simulink model "BLDC_dq_Control_Gradual"  (R2021a)
settings: Solver=FixedStepAuto  StartTime=0.0  StopTime=12  FixedStep=0.000002  RelTol=1e-3
model workspace (MAT data in the model file):
  Tl = 3
undefined symbols (not defined in the file): sigbuilder_block
libraries: pid_lib x9, spsMosfetLib x6, spsVoltageMeasurementLib x3, simulink x2, spsDCVoltageSourceLib x1, spspowerguiLib x1
(part 1 of 2)
settings Model: Creator=raca  LastModifiedBy=headl
settings SolverCC: AlgebraicLoopSolver=TrustRegion
settings DataIOCC: ReturnWorkspaceOutputs=off
settings DebuggingCC: SFMachineParentedDataDiag=warning  ArithmeticOperatorsInVariantConditions=warning
settings SFSimCC: SimUseLocalCustomCode=off  CustomCodeUndefinedFunction=UseInterfaceOnly
settings RTWCC: RTWUseLocalCustomCode=off
settings CodeAppCC: StateflowObjectComments=on

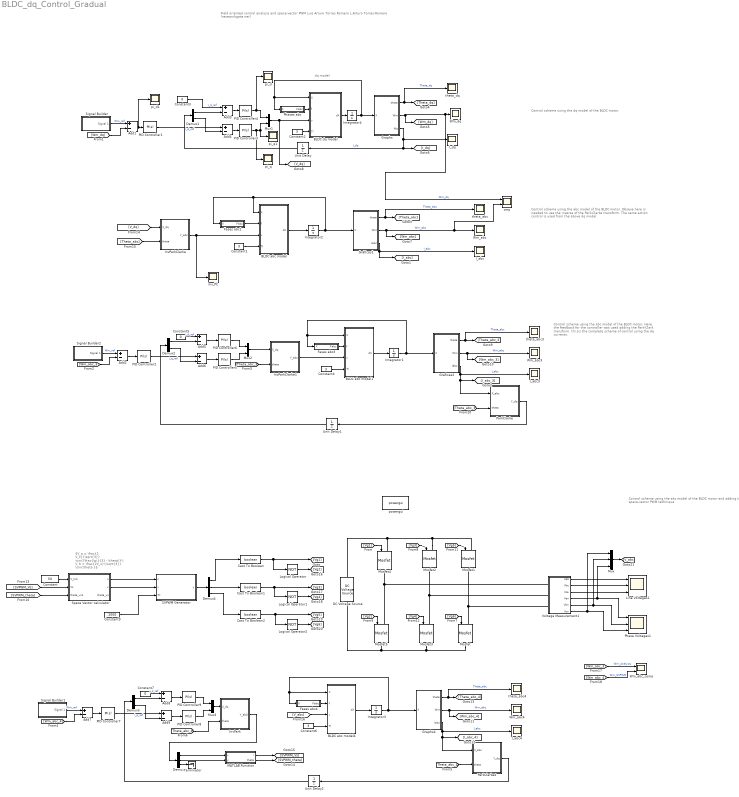
== system BLDC_dq_Control_Gradual ==
  note: Control scheme using the dq model of the BLDC motor.
  note: Field oriented control analysis and space-vector PWM
      | Luis Arturo Torres Romero
      |
      | L.Arturo Torres-Romero (researchgate.net)
  note: $V_a = \frac{2 V_s}{\sqrt{3}} \sin{(\frac{\pi}{3} - \theta)}\\ V_b = \frac{2V_s}{\sqrt{3}} \sin{\theta }$
  note: dq model
  note: Control scheme using the abc model of the BLDC motor.
      |
      | Obseve here is needed to use the inverse of the Park-Clarke transform. The same action control is used from the above dq model.
  note: Control scheme using the abc model of the BLDC motor.
      |
      | Here, the feedback for the controller was used adding the Park-Clark transform. thi sis the complete scheme of control using the dq currents.
  note: Control scheme using the abc model of the BLDC motor and adding the space-vector PWM technique
  Add{1..9} (9 alike) : Sum  Inputs=+-
  BLDC abc model : MATLAB Function  TreatAsAtomicUnit=on
  BLDC abc model1 : MATLAB Function  TreatAsAtomicUnit=on
  BLDC abc model4 : MATLAB Function  TreatAsAtomicUnit=on
  BLDC dq model : MATLAB Function  TreatAsAtomicUnit=on
  Cast To Boolean : DataTypeConversion  OutDataTypeStr=boolean
  Cast To Boolean1 : DataTypeConversion  OutDataTypeStr=boolean
  Cast To Boolean2 : DataTypeConversion  OutDataTypeStr=boolean
  Constant : Constant  Value=50
  Constant{1..2,4,6} (4 alike) : Constant  Value=3
  Constant3 : Constant  Value=0
  Constant5 : Constant  Value=0
  Constant7 : Constant  Value=0
  Constant9 : Constant  Value=2000
  DC Voltage Source : spsDCVoltageSourceLib/DC Voltage Source  Amplitude=50  Measurements=None
  Demux : Demux  Outputs=3
  Demux1 : Demux  Outputs=2
  Demux2 : Demux  Outputs=2
  Demux3 : Demux  Outputs=2
  Demux4 : Demux  Outputs=3
  Fases abc1 : MATLAB Function  TreatAsAtomicUnit=on
  Fases abc3 : MATLAB Function  TreatAsAtomicUnit=on
  Fases abc4 : MATLAB Function  TreatAsAtomicUnit=on
  Graphs : MATLAB Function  TreatAsAtomicUnit=on
  Graphs4 : MATLAB Function  TreatAsAtomicUnit=on
  Gráficas1 : MATLAB Function  TreatAsAtomicUnit=on
  Gráficas2 : MATLAB Function  TreatAsAtomicUnit=on
  I_abc : Scope
  I_abc3 : Scope
  I_abc4 : Scope
  I_dq : Scope
  Integrator1 : Integrator  InitialCondition=[0;0;0;0.1;0.1]
  Integrator2 : Integrator  InitialCondition=[0;0;0;0.1;0.1]
  Integrator3 : Integrator  InitialCondition=[0;0;0;0.1;0.1]
  Integrator4 : Integrator  InitialCondition=[0;0;0.1;0.1]
  InvPark : MATLAB Function  TreatAsAtomicUnit=on
  InvParkClarke : MATLAB Function  TreatAsAtomicUnit=on
  InvParkClarke1 : MATLAB Function  TreatAsAtomicUnit=on
  Line Voltages1 : Scope  NumInputPorts=3
  Logical Operator : Logic  Operator=NOT  IconShape=distinctive  AllPortsSameDT=off  OutDataTypeStr=boolean
  Logical Operator1 : Logic  Operator=NOT  IconShape=distinctive  AllPortsSameDT=off  OutDataTypeStr=boolean
  Logical Operator2 : Logic  Operator=NOT  IconShape=distinctive  AllPortsSameDT=off  OutDataTypeStr=boolean
  MATLAB Function : MATLAB Function  TreatAsAtomicUnit=on
  Mosfet{,1..5} (6 alike) : spsMosfetLib/Mosfet  Ron=0.1  Lon=0  Rd=0.01  Vfd=0  IC=0  Rs=1e5  Cs=inf  Measurements=off
  Mux : Mux  Inputs=3
  Mux1 : Mux  Inputs=2
  Mux2 : Mux  Inputs=2
  Mux3 : Mux  Inputs=2
  PID Controller1 : pid_lib/PID Controller  Controller=PI  Form=Parallel  TimeDomain=Continuous-time  UseExternalTs=off  SampleTime=-1  IntegratorMethod=Forward Euler  FilterMethod=Forward Euler  ControllerParametersSource=internal  P=-0.39820378606854  I=-44.4991237925307  D=0  UseFilter=on  N=100  TunerSelectOption=Transfer Function Based (PID Tuner App)  InitialConditionSource=internal  InitialConditionForIntegrator=0  InitialConditionForFilter=0  DifferentiatorICPrevScaledInput=0  ExternalReset=none  TrackingMode=off  Kt=1  LimitOutput=off  SatLimitsSource=internal  UpperSaturationLimit=inf  LowerSaturationLimit=-inf  LinearizeAsGain=on  AntiWindupMode=none  Kb=1  POutMin=[]  POutMax=[]  IOutMin=[]  IOutMax=[]  DOutMin=[]  DOutMax=[]  NOutMin=[]  NOutMax=[]  SumOutMin=[]  SumOutMax=[]  SaturationOutMin=[]  SaturationOutMax=[]  PParamMin=[]  PParamMax=[]  IParamMin=[]  IParamMax=[]  DParamMin=[]  DParamMax=[]  NParamMin=[]  NParamMax=[]  KbParamMin=[]  KbParamMax=[]  KtParamMin=[]  KtParamMax=[]  KbOutMin=[]  KbOutMax=[]  KtOutMin=[]  KtOutMax=[]  IntegratorOutMin=[]  IntegratorOutMax=[]  FilterOutMin=[]  FilterOutMax=[]  SumI1OutMin=[]  SumI1OutMax=[]  SumI2OutMin=[]  SumI2OutMax=[]  SumI3OutMin=[]  SumI3OutMax=[]  SumI4OutMin=[]  SumI4OutMax=[]  SumDOutMin=[]  SumDOutMax=[]  DifferentiatorOutMin=[]  DifferentiatorOutMax=[]  FilterDiffOutCoefMin=[]  FilterDiffOutCoefMax=[]  ReciprocalOutMin=[]  ReciprocalOutMax=[]  SumDenOutMin=[]  SumDenOutMax=[]  SumNumOutMin=[]  SumNumOutMax=[]  DivideOutMin=[]  DivideOutMax=[]  UdiffTsProdOutMin=[]  UdiffTsProdOutMax=[]  NTsProdOutMin=[]  NTsProdOutMax=[]  UintegralTsProdOutMin=[]  UintegralTsProdOutMax=[]  UngainTsProdOutMin=[]  UngainTsProdOutMax=[]  IntegratorContinuousStateAttributes=''  IntegratorStateMustResolveToSignalObject=off  IntegratorRTWStateStorageClass=Auto  FilterContinuousStateAttributes=''  FilterStateMustResolveToSignalObject=off  FilterRTWStateStorageClass=Auto  ParallelPVariant=InternalParameters  IdealPVariant=Disabled  IVariant=InternalParameters  DVariant=Disabled  IntegratorVariant=Continuous  SatVariant=Disabled  AWVariant=Passthrough  PCopyVariant=Disabled  TRVariant=Disabled  FdbkBlocksVariant=Forward  IdealPFdbkVariant=Disabled  SatFdbkVariant=Disabled  DerivativeFilterVariant=Disabled  NVariant=Disabled  NCopyVariant=Disabled_SignalSpec  FilterICVariant=Disabled  IntegratorICVariant=InternalICs  ExternalResetVariant=Disabled  TRSumVariant=Passthrough  SumFdbkVariant=Disabled  SumVariant=Sum_PI  TsampFilterVariant=InternalTs  TsampNgainVariant=Passthrough  TsampIntegralVariant=Passthrough  ExternalSaturationOutDataTypeStr=Inherit: Same as second input
  PID Controller2 : pid_lib/PID Controller  Controller=PI  Form=Parallel  TimeDomain=Continuous-time  UseExternalTs=off  SampleTime=-1  IntegratorMethod=Forward Euler  FilterMethod=Forward Euler  ControllerParametersSource=internal  P=-0.39820378606854  I=-44.4991237925307  D=0  UseFilter=on  N=100  TunerSelectOption=Transfer Function Based (PID Tuner App)  InitialConditionSource=internal  InitialConditionForIntegrator=0  InitialConditionForFilter=0  DifferentiatorICPrevScaledInput=0  ExternalReset=none  TrackingMode=off  Kt=1  LimitOutput=off  SatLimitsSource=internal  UpperSaturationLimit=inf  LowerSaturationLimit=-inf  LinearizeAsGain=on  AntiWindupMode=none  Kb=1  POutMin=[]  POutMax=[]  IOutMin=[]  IOutMax=[]  DOutMin=[]  DOutMax=[]  NOutMin=[]  NOutMax=[]  SumOutMin=[]  SumOutMax=[]  SaturationOutMin=[]  SaturationOutMax=[]  PParamMin=[]  PParamMax=[]  IParamMin=[]  IParamMax=[]  DParamMin=[]  DParamMax=[]  NParamMin=[]  NParamMax=[]  KbParamMin=[]  KbParamMax=[]  KtParamMin=[]  KtParamMax=[]  KbOutMin=[]  KbOutMax=[]  KtOutMin=[]  KtOutMax=[]  IntegratorOutMin=[]  IntegratorOutMax=[]  FilterOutMin=[]  FilterOutMax=[]  SumI1OutMin=[]  SumI1OutMax=[]  SumI2OutMin=[]  SumI2OutMax=[]  SumI3OutMin=[]  SumI3OutMax=[]  SumI4OutMin=[]  SumI4OutMax=[]  SumDOutMin=[]  SumDOutMax=[]  DifferentiatorOutMin=[]  DifferentiatorOutMax=[]  FilterDiffOutCoefMin=[]  FilterDiffOutCoefMax=[]  ReciprocalOutMin=[]  ReciprocalOutMax=[]  SumDenOutMin=[]  SumDenOutMax=[]  SumNumOutMin=[]  SumNumOutMax=[]  DivideOutMin=[]  DivideOutMax=[]  UdiffTsProdOutMin=[]  UdiffTsProdOutMax=[]  NTsProdOutMin=[]  NTsProdOutMax=[]  UintegralTsProdOutMin=[]  UintegralTsProdOutMax=[]  UngainTsProdOutMin=[]  UngainTsProdOutMax=[]  IntegratorContinuousStateAttributes=''  IntegratorStateMustResolveToSignalObject=off  IntegratorRTWStateStorageClass=Auto  FilterContinuousStateAttributes=''  FilterStateMustResolveToSignalObject=off  FilterRTWStateStorageClass=Auto  ParallelPVariant=InternalParameters  IdealPVariant=Disabled  IVariant=InternalParameters  DVariant=Disabled  IntegratorVariant=Continuous  SatVariant=Disabled  AWVariant=Passthrough  PCopyVariant=Disabled  TRVariant=Disabled  FdbkBlocksVariant=Forward  IdealPFdbkVariant=Disabled  SatFdbkVariant=Disabled  DerivativeFilterVariant=Disabled  NVariant=Disabled  NCopyVariant=Disabled_SignalSpec  FilterICVariant=Disabled  IntegratorICVariant=InternalICs  ExternalResetVariant=Disabled  TRSumVariant=Passthrough  SumFdbkVariant=Disabled  SumVariant=Sum_PI  TsampFilterVariant=InternalTs  TsampNgainVariant=Passthrough  TsampIntegralVariant=Passthrough  ExternalSaturationOutDataTypeStr=Inherit: Same as second input
  PID Controller3 : pid_lib/PID Controller  Controller=PI  Form=Parallel  TimeDomain=Continuous-time  UseExternalTs=off  SampleTime=-1  IntegratorMethod=Forward Euler  FilterMethod=Forward Euler  ControllerParametersSource=internal  P=70  I=0.3  D=-0.000363636535687767  UseFilter=on  N=1.72044274974478  TunerSelectOption=Transfer Function Based (PID Tuner App)  InitialConditionSource=internal  InitialConditionForIntegrator=0  InitialConditionForFilter=0  DifferentiatorICPrevScaledInput=0  ExternalReset=none  TrackingMode=off  Kt=1  LimitOutput=off  SatLimitsSource=internal  UpperSaturationLimit=inf  LowerSaturationLimit=-inf  LinearizeAsGain=on  AntiWindupMode=none  Kb=1  POutMin=[]  POutMax=[]  IOutMin=[]  IOutMax=[]  DOutMin=[]  DOutMax=[]  NOutMin=[]  NOutMax=[]  SumOutMin=[]  SumOutMax=[]  SaturationOutMin=[]  SaturationOutMax=[]  PParamMin=[]  PParamMax=[]  IParamMin=[]  IParamMax=[]  DParamMin=[]  DParamMax=[]  NParamMin=[]  NParamMax=[]  KbParamMin=[]  KbParamMax=[]  KtParamMin=[]  KtParamMax=[]  KbOutMin=[]  KbOutMax=[]  KtOutMin=[]  KtOutMax=[]  IntegratorOutMin=[]  IntegratorOutMax=[]  FilterOutMin=[]  FilterOutMax=[]  SumI1OutMin=[]  SumI1OutMax=[]  SumI2OutMin=[]  SumI2OutMax=[]  SumI3OutMin=[]  SumI3OutMax=[]  SumI4OutMin=[]  SumI4OutMax=[]  SumDOutMin=[]  SumDOutMax=[]  DifferentiatorOutMin=[]  DifferentiatorOutMax=[]  FilterDiffOutCoefMin=[]  FilterDiffOutCoefMax=[]  ReciprocalOutMin=[]  ReciprocalOutMax=[]  SumDenOutMin=[]  SumDenOutMax=[]  SumNumOutMin=[]  SumNumOutMax=[]  DivideOutMin=[]  DivideOutMax=[]  UdiffTsProdOutMin=[]  UdiffTsProdOutMax=[]  NTsProdOutMin=[]  NTsProdOutMax=[]  UintegralTsProdOutMin=[]  UintegralTsProdOutMax=[]  UngainTsProdOutMin=[]  UngainTsProdOutMax=[]  IntegratorContinuousStateAttributes=''  IntegratorStateMustResolveToSignalObject=off  IntegratorRTWStateStorageClass=Auto  FilterContinuousStateAttributes=''  FilterStateMustResolveToSignalObject=off  FilterRTWStateStorageClass=Auto  ParallelPVariant=InternalParameters  IdealPVariant=Disabled  IVariant=InternalParameters  DVariant=Disabled  IntegratorVariant=Continuous  SatVariant=Disabled  AWVariant=Passthrough  PCopyVariant=Disabled  TRVariant=Disabled  FdbkBlocksVariant=Forward  IdealPFdbkVariant=Disabled  SatFdbkVariant=Disabled  DerivativeFilterVariant=Disabled  NVariant=Disabled  NCopyVariant=Disabled_SignalSpec  FilterICVariant=Disabled  IntegratorICVariant=InternalICs  ExternalResetVariant=Disabled  TRSumVariant=Passthrough  SumFdbkVariant=Disabled  SumVariant=Sum_PI  TsampFilterVariant=InternalTs  TsampNgainVariant=Passthrough  TsampIntegralVariant=Passthrough  ExternalSaturationOutDataTypeStr=Inherit: Same as second input
  PID Controller4 : pid_lib/PID Controller  Controller=PI  Form=Parallel  TimeDomain=Continuous-time  UseExternalTs=off  SampleTime=-1  IntegratorMethod=Forward Euler  FilterMethod=Forward Euler  ControllerParametersSource=internal  P=70  I=0.3  D=-6.74177637974606e-05  UseFilter=on  N=1209.06435302465  TunerSelectOption=Transfer Function Based (PID Tuner App)  InitialConditionSource=internal  InitialConditionForIntegrator=0  InitialConditionForFilter=0  DifferentiatorICPrevScaledInput=0  ExternalReset=none  TrackingMode=off  Kt=1  LimitOutput=off  SatLimitsSource=internal  UpperSaturationLimit=inf  LowerSaturationLimit=-inf  LinearizeAsGain=on  AntiWindupMode=none  Kb=1  POutMin=[]  POutMax=[]  IOutMin=[]  IOutMax=[]  DOutMin=[]  DOutMax=[]  NOutMin=[]  NOutMax=[]  SumOutMin=[]  SumOutMax=[]  SaturationOutMin=[]  SaturationOutMax=[]  PParamMin=[]  PParamMax=[]  IParamMin=[]  IParamMax=[]  DParamMin=[]  DParamMax=[]  NParamMin=[]  NParamMax=[]  KbParamMin=[]  KbParamMax=[]  KtParamMin=[]  KtParamMax=[]  KbOutMin=[]  KbOutMax=[]  KtOutMin=[]  KtOutMax=[]  IntegratorOutMin=[]  IntegratorOutMax=[]  FilterOutMin=[]  FilterOutMax=[]  SumI1OutMin=[]  SumI1OutMax=[]  SumI2OutMin=[]  SumI2OutMax=[]  SumI3OutMin=[]  SumI3OutMax=[]  SumI4OutMin=[]  SumI4OutMax=[]  SumDOutMin=[]  SumDOutMax=[]  DifferentiatorOutMin=[]  DifferentiatorOutMax=[]  FilterDiffOutCoefMin=[]  FilterDiffOutCoefMax=[]  ReciprocalOutMin=[]  ReciprocalOutMax=[]  SumDenOutMin=[]  SumDenOutMax=[]  SumNumOutMin=[]  SumNumOutMax=[]  DivideOutMin=[]  DivideOutMax=[]  UdiffTsProdOutMin=[]  UdiffTsProdOutMax=[]  NTsProdOutMin=[]  NTsProdOutMax=[]  UintegralTsProdOutMin=[]  UintegralTsProdOutMax=[]  UngainTsProdOutMin=[]  UngainTsProdOutMax=[]  IntegratorContinuousStateAttributes=''  IntegratorStateMustResolveToSignalObject=off  IntegratorRTWStateStorageClass=Auto  FilterContinuousStateAttributes=''  FilterStateMustResolveToSignalObject=off  FilterRTWStateStorageClass=Auto  ParallelPVariant=InternalParameters  IdealPVariant=Disabled  IVariant=InternalParameters  DVariant=Disabled  IntegratorVariant=Continuous  SatVariant=Disabled  AWVariant=Passthrough  PCopyVariant=Disabled  TRVariant=Disabled  FdbkBlocksVariant=Forward  IdealPFdbkVariant=Disabled  SatFdbkVariant=Disabled  DerivativeFilterVariant=Disabled  NVariant=Disabled  NCopyVariant=Disabled_SignalSpec  FilterICVariant=Disabled  IntegratorICVariant=InternalICs  ExternalResetVariant=Disabled  TRSumVariant=Passthrough  SumFdbkVariant=Disabled  SumVariant=Sum_PI  TsampFilterVariant=InternalTs  TsampNgainVariant=Passthrough  TsampIntegralVariant=Passthrough  ExternalSaturationOutDataTypeStr=Inherit: Same as second input
  PID Controller{5..6,8..9} (4 alike) : pid_lib/PID Controller  Controller=PI  Form=Parallel  TimeDomain=Continuous-time  UseExternalTs=off  SampleTime=-1  IntegratorMethod=Forward Euler  FilterMethod=Forward Euler  ControllerParametersSource=internal  P=70  I=0.3  D=0  UseFilter=on  N=100  TunerSelectOption=Transfer Function Based (PID Tuner App)  InitialConditionSource=internal  InitialConditionForIntegrator=0  InitialConditionForFilter=0  DifferentiatorICPrevScaledInput=0  ExternalReset=none  TrackingMode=off  Kt=1  LimitOutput=off  SatLimitsSource=internal  UpperSaturationLimit=inf  LowerSaturationLimit=-inf  LinearizeAsGain=on  AntiWindupMode=none  Kb=1  POutMin=[]  POutMax=[]  IOutMin=[]  IOutMax=[]  DOutMin=[]  DOutMax=[]  NOutMin=[]  NOutMax=[]  SumOutMin=[]  SumOutMax=[]  SaturationOutMin=[]  SaturationOutMax=[]  PParamMin=[]  PParamMax=[]  IParamMin=[]  IParamMax=[]  DParamMin=[]  DParamMax=[]  NParamMin=[]  NParamMax=[]  KbParamMin=[]  KbParamMax=[]  KtParamMin=[]  KtParamMax=[]  KbOutMin=[]  KbOutMax=[]  KtOutMin=[]  KtOutMax=[]  IntegratorOutMin=[]  IntegratorOutMax=[]  FilterOutMin=[]  FilterOutMax=[]  SumI1OutMin=[]  SumI1OutMax=[]  SumI2OutMin=[]  SumI2OutMax=[]  SumI3OutMin=[]  SumI3OutMax=[]  SumI4OutMin=[]  SumI4OutMax=[]  SumDOutMin=[]  SumDOutMax=[]  DifferentiatorOutMin=[]  DifferentiatorOutMax=[]  FilterDiffOutCoefMin=[]  FilterDiffOutCoefMax=[]  ReciprocalOutMin=[]  ReciprocalOutMax=[]  SumDenOutMin=[]  SumDenOutMax=[]  SumNumOutMin=[]  SumNumOutMax=[]  DivideOutMin=[]  DivideOutMax=[]  UdiffTsProdOutMin=[]  UdiffTsProdOutMax=[]  NTsProdOutMin=[]  NTsProdOutMax=[]  UintegralTsProdOutMin=[]  UintegralTsProdOutMax=[]  UngainTsProdOutMin=[]  UngainTsProdOutMax=[]  IntegratorContinuousStateAttributes=''  IntegratorStateMustResolveToSignalObject=off  IntegratorRTWStateStorageClass=Auto  FilterContinuousStateAttributes=''  FilterStateMustResolveToSignalObject=off  FilterRTWStateStorageClass=Auto  ParallelPVariant=InternalParameters  IdealPVariant=Disabled  IVariant=InternalParameters  DVariant=Disabled  IntegratorVariant=Continuous  SatVariant=Disabled  AWVariant=Passthrough  PCopyVariant=Disabled  TRVariant=Disabled  FdbkBlocksVariant=Forward  IdealPFdbkVariant=Disabled  SatFdbkVariant=Disabled  DerivativeFilterVariant=Disabled  NVariant=Disabled  NCopyVariant=Disabled_SignalSpec  FilterICVariant=Disabled  IntegratorICVariant=InternalICs  ExternalResetVariant=Disabled  TRSumVariant=Passthrough  SumFdbkVariant=Disabled  SumVariant=Sum_PI  TsampFilterVariant=InternalTs  TsampNgainVariant=Passthrough  TsampIntegralVariant=Passthrough  ExternalSaturationOutDataTypeStr=Inherit: Same as second input
  PID Controller7 : pid_lib/PID Controller  Controller=PI  Form=Parallel  TimeDomain=Continuous-time  UseExternalTs=off  SampleTime=-1  IntegratorMethod=Forward Euler  FilterMethod=Forward Euler  ControllerParametersSource=internal  P=-0.39820378606854  I=-44.4991237925307  D=0  UseFilter=on  N=100  TunerSelectOption=Transfer Function Based (PID Tuner App)  InitialConditionSource=internal  InitialConditionForIntegrator=0  InitialConditionForFilter=0  DifferentiatorICPrevScaledInput=0  ExternalReset=none  TrackingMode=off  Kt=1  LimitOutput=off  SatLimitsSource=internal  UpperSaturationLimit=inf  LowerSaturationLimit=-inf  LinearizeAsGain=on  AntiWindupMode=none  Kb=1  POutMin=[]  POutMax=[]  IOutMin=[]  IOutMax=[]  DOutMin=[]  DOutMax=[]  NOutMin=[]  NOutMax=[]  SumOutMin=[]  SumOutMax=[]  SaturationOutMin=[]  SaturationOutMax=[]  PParamMin=[]  PParamMax=[]  IParamMin=[]  IParamMax=[]  DParamMin=[]  DParamMax=[]  NParamMin=[]  NParamMax=[]  KbParamMin=[]  KbParamMax=[]  KtParamMin=[]  KtParamMax=[]  KbOutMin=[]  KbOutMax=[]  KtOutMin=[]  KtOutMax=[]  IntegratorOutMin=[]  IntegratorOutMax=[]  FilterOutMin=[]  FilterOutMax=[]  SumI1OutMin=[]  SumI1OutMax=[]  SumI2OutMin=[]  SumI2OutMax=[]  SumI3OutMin=[]  SumI3OutMax=[]  SumI4OutMin=[]  SumI4OutMax=[]  SumDOutMin=[]  SumDOutMax=[]  DifferentiatorOutMin=[]  DifferentiatorOutMax=[]  FilterDiffOutCoefMin=[]  FilterDiffOutCoefMax=[]  ReciprocalOutMin=[]  ReciprocalOutMax=[]  SumDenOutMin=[]  SumDenOutMax=[]  SumNumOutMin=[]  SumNumOutMax=[]  DivideOutMin=[]  DivideOutMax=[]  UdiffTsProdOutMin=[]  UdiffTsProdOutMax=[]  NTsProdOutMin=[]  NTsProdOutMax=[]  UintegralTsProdOutMin=[]  UintegralTsProdOutMax=[]  UngainTsProdOutMin=[]  UngainTsProdOutMax=[]  IntegratorContinuousStateAttributes=''  IntegratorStateMustResolveToSignalObject=off  IntegratorRTWStateStorageClass=Auto  FilterContinuousStateAttributes=''  FilterStateMustResolveToSignalObject=off  FilterRTWStateStorageClass=Auto  ParallelPVariant=InternalParameters  IdealPVariant=Disabled  IVariant=InternalParameters  DVariant=Disabled  IntegratorVariant=Continuous  SatVariant=Disabled  AWVariant=Passthrough  PCopyVariant=Disabled  TRVariant=Disabled  FdbkBlocksVariant=Forward  IdealPFdbkVariant=Disabled  SatFdbkVariant=Disabled  DerivativeFilterVariant=Disabled  NVariant=Disabled  NCopyVariant=Disabled_SignalSpec  FilterICVariant=Disabled  IntegratorICVariant=InternalICs  ExternalResetVariant=Disabled  TRSumVariant=Passthrough  SumFdbkVariant=Disabled  SumVariant=Sum_PI  TsampFilterVariant=InternalTs  TsampNgainVariant=Passthrough  TsampIntegralVariant=Passthrough  ExternalSaturationOutDataTypeStr=Inherit: Same as second input
  ParkClarke : MATLAB Function  TreatAsAtomicUnit=on
  ParkClarke4 : MATLAB Function  TreatAsAtomicUnit=on
  Phase Voltages1 : Scope  NumInputPorts=3
  Phases abc : MATLAB Function  TreatAsAtomicUnit=on
  SVPWM Generator : Subsystem
  Signal Builder : Subsystem  Tag=STV Subsys  LoadFcn=sigbuilder_block('load');  StartFcn=sigbuilder_block('start');  StopFcn=sigbuilder_block('stop');  ClipboardFcn=sigbuilder_block('clipboard');  mask(Sigbuilder block){tuvar=[0:10]}
      mask help: Simulink:masks:SigbuilderBlock_MD
      mask init:
      | if ~strcmp(get_param(bdroot(gcbh),'SimulationStatus'),'stopped') tuvar = sigbuilder_block('maskInit'); end
      settings: CopyFcn=sigbuilder_block('copy');  DeleteFcn=sigbuilder_block('delete');  ModelCloseFcn=sigbuilder_block('modelClose');  PreSaveFcn=sigbuilder_block('preSave');  PauseFcn=sigbuilder_block('pause');  ContinueFcn=sigbuilder_block('continue');  NameChangeFcn=sigbuilder_block('namechange');  OpenFcn=sigbuilder_block('open',[0 30 1152 561.6 ]);  CloseFcn=sigbuilder_block('close');
      mask Display: plot(0, 0, 100, 100,[2, 2, 32, 32, 2], [68, 8, 8, 68, 68],[32, 2], [38, 38], [32, 19, 2],[53, 60, 44], [32, 17, 17, 2],[16, 16, 31, 31]);txt = getActiveGroup(gcbh);text(2, 100, txt,'verticalAlignment', 'top');
  Signal Builder1 : Subsystem  Tag=STV Subsys  LoadFcn=sigbuilder_block('load');  StartFcn=sigbuilder_block('start');  StopFcn=sigbuilder_block('stop');  ClipboardFcn=sigbuilder_block('clipboard');  mask(Sigbuilder block){tuvar=[0:10]}
      mask help: Simulink:masks:SigbuilderBlock_MD
      mask init:
      | if ~strcmp(get_param(bdroot(gcbh),'SimulationStatus'),'stopped') tuvar = sigbuilder_block('maskInit'); end
      settings: CopyFcn=sigbuilder_block('copy');  DeleteFcn=sigbuilder_block('delete');  ModelCloseFcn=sigbuilder_block('modelClose');  PreSaveFcn=sigbuilder_block('preSave');  PauseFcn=sigbuilder_block('pause');  ContinueFcn=sigbuilder_block('continue');  NameChangeFcn=sigbuilder_block('namechange');  OpenFcn=sigbuilder_block('open',[5.4 30 1141.2 522.6 ]);  CloseFcn=sigbuilder_block('close');
      mask Display: plot(0, 0, 100, 100,[2, 2, 32, 32, 2], [68, 8, 8, 68, 68],[32, 2], [38, 38], [32, 19, 2],[53, 60, 44], [32, 17, 17, 2],[16, 16, 31, 31]);txt = getActiveGroup(gcbh);text(2, 100, txt,'verticalAlignment', 'top');
  Signal Builder2 : Subsystem  Tag=STV Subsys  LoadFcn=sigbuilder_block('load');  StartFcn=sigbuilder_block('start');  StopFcn=sigbuilder_block('stop');  ClipboardFcn=sigbuilder_block('clipboard');  mask(Sigbuilder block){tuvar=[0:10]}
      mask help: Simulink:masks:SigbuilderBlock_MD
      mask init:
      | if ~strcmp(get_param(bdroot(gcbh),'SimulationStatus'),'stopped') tuvar = sigbuilder_block('maskInit'); end
      settings: CopyFcn=sigbuilder_block('copy');  DeleteFcn=sigbuilder_block('delete');  ModelCloseFcn=sigbuilder_block('modelClose');  PreSaveFcn=sigbuilder_block('preSave');  PauseFcn=sigbuilder_block('pause');  ContinueFcn=sigbuilder_block('continue');  NameChangeFcn=sigbuilder_block('namechange');  OpenFcn=sigbuilder_block('open',[0 30 1152 561.6 ]);  CloseFcn=sigbuilder_block('close');
      mask Display: plot(0, 0, 100, 100,[2, 2, 32, 32, 2], [68, 8, 8, 68, 68],[32, 2], [38, 38], [32, 19, 2],[53, 60, 44], [32, 17, 17, 2],[16, 16, 31, 31]);txt = getActiveGroup(gcbh);text(2, 100, txt,'verticalAlignment', 'top');
  Space Vector calculator : MATLAB Function  TreatAsAtomicUnit=on
  Terminator : Terminator
  Unit Delay : UnitDelay  SampleTime=-1  HasFrameUpgradeWarning=on
  Unit Delay1 : UnitDelay  SampleTime=-1  HasFrameUpgradeWarning=on
  Unit Delay2 : UnitDelay  SampleTime=-1  HasFrameUpgradeWarning=on
  Voltage Measurement1 : Subsystem
  Wm_abc : Scope
  Wm_abc3 : Scope
  Wm_abc4 : Scope
  Wm_abc_comp : Scope  NumInputPorts=2
  Wm_dq : Scope
  cmp : Scope  NumInputPorts=2
  inv_PC : Scope
  pi_d : Scope
  pi_d1 : Scope
  pi_q : Scope
  pi_q1 : Scope
  powergui : spspowerguiLib/powergui  Priority=1  SimulationMode=Discrete  SampleTime=2e-6  frequency=60  Iterations=50  frequencyindice=0  Pbase=100e6  ErrMax=1e-4  UnitsV=kV  UnitsW=MW  buscounter=0  FunctionMessages=off  echomessages=off  EnableUseOfTLC=off  CurrentSourceSwitches=off  DisableSnubberDevices=off  DisableRonSwitches=off  DisableVfSwitches=off  DisplayEquations=off  AutomaticDiscreteSolvers=off  SolverType=Tustin/Backward Euler (TBE)  Interpol=off  ExternalGateDelay=off  methode=off  Ts=100  x0status=blocks  SPID=off  SwTol=0  HookPort=off  NonlinearTolerance=1e-4  nMaxIteration=100  ContinueOnMaxIteration=off  RestoreLinks=warning  ResistiveCurrentMeasurement=off  Frange=[0:2:500]  Ylog=off  Xlog=on  ShowGrid=off  save=off  variable=ZData  structure=ScopeData3  ZoomFFT=off  StartTime=0.04  cycles=1  DisplayStyle=1  fundamental=50  FreqAxis=off  MaxFrequency=2000  frequencyindicesteady=1  RmsSteady=1  display=off
  theta_abc : Scope
  theta_abc3 : Scope
  theta_abc4 : Scope
  theta_dq : Scope
  wires:
  Graphs/1(theta) -> [Theta_dq], theta_dq/1  "Theta_dq"
  BLDC dq model/1(dX) -> Integrator4/1
  Integrator4/1 -> Graphs/1(X), BLDC dq model/1(X), Phases abc/1(X)
  Graphs/3(Idq) -> [I_dq], Unit Delay/1, I_dq/1  "I_dq"
  Graphs/2(Wm) -> cmp/1, Wm_dq/1, [Wm_dq]  "Wm_dq"
  Phases abc/1(Fabc) -> BLDC dq model/2(f)
  Constant2/1 -> BLDC dq model/4(Tl)
  Add4/1 -> PID Controller3/1
  Add3/1 -> PID Controller4/1
  Demux1/2 -> Add4/2
  Demux1/1 -> Add3/2
  PID Controller4/1 -> pi_d/1, Mux1/1
  PID Controller3/1 -> pi_q/1, Mux1/2, pi_q1/1
  Mux1/1 -> [V_dq], BLDC dq model/3(v)
  Unit Delay/1 -> Demux1/1
  Add1/1 -> pi_d1/1, PID Controller1/1
  [Wm_dq] -> Add1/2
  Signal Builder/1(Signal 1) -> Add1/1  "Wm_ref"
  BLDC abc model/1(dX) -> Integrator2/1
  Gráficas1/3(Iabc) -> [I_abc], I_abc/1  "I_abc"
  Gráficas1/1(theta) -> theta_abc/1, [Theta_abc]  "Theta_abc"
  InvParkClarke/1(Y_abc) -> inv_PC/1, BLDC abc model/3(v)
  Constant1/1 -> BLDC abc model/4(Tl)
  Fases abc1/1(Fabc) -> BLDC abc model/2(f)
  Integrator2/1 -> Gráficas1/1(X), Fases abc1/1(X), BLDC abc model/1(X)
  Gráficas1/2(Wm) -> [Wm_abc], cmp/2, Wm_abc/1  "Wm_abc"
  [V_dq] -> InvParkClarke/1(X_dq)
  [Theta_abc] -> InvParkClarke/2(theta)
  Constant3/1 -> Add3/1  "i_d_ref"
  PID Controller1/1 -> Add4/1  "i_d_ref"
  Demux2/2 -> Add6/2
  PID Controller6/1 -> Mux2/1
  Unit Delay1/1 -> Demux2/1
  [Wm_abc_3] -> Add2/2
  Demux2/1 -> Add5/2
  Add5/1 -> PID Controller6/1
  Integrator1/1 -> Gráficas2/1(X), BLDC abc model1/1(X), Fases abc3/1(X)
  PID Controller5/1 -> Mux2/2
  Constant5/1 -> Add5/1  "i_d_ref"
  [Theta_abc_3] -> ParkClarke/2(theta)
  Signal Builder2/1(Signal 1) -> Add2/1  "Wm_ref"
  ParkClarke/1(Y_dq) -> Unit Delay1/1
  Add2/1 -> PID Controller2/1
  PID Controller2/1 -> Add6/1  "i_q_ref"
  InvParkClarke1/1(Y_abc) -> BLDC abc model1/3(v)
  Add6/1 -> PID Controller5/1
  Fases abc3/1(Fabc) -> BLDC abc model1/2(f)
  Mux2/1 -> InvParkClarke1/1(X_dq)
  [Theta_abc_3] -> InvParkClarke1/2(theta)
  BLDC abc model1/1(dX) -> Integrator1/1
  Gráficas2/1(theta) -> theta_abc3/1, [Theta_abc_3]  "Theta_abc"
  Gráficas2/2(Wm) -> [Wm_abc_3], Wm_abc3/1  "Wm_abc"
  Constant4/1 -> BLDC abc model1/4(Tl)
  Gráficas2/3(Iabc) -> [I_abc_3], ParkClarke/1(X_abc), I_abc3/1  "I_abc"
  Fases abc4/1(Fabc) -> BLDC abc model4/2(f)
  Graphs4/3(Iabc) -> [I_abc_4], ParkClarke4/1(X_abc), I_abc4/1  "I_abc"
  Constant6/1 -> BLDC abc model4/4(Tl)
  Graphs4/1(theta) -> theta_abc4/1, [Theta_abc_4]  "Theta_abc"
  Demux3/2 -> Add9/2
  Signal Builder1/1(Signal 1) -> Add7/1  "Wm_ref"
  Graphs4/2(Wm) -> [Wm_abc_4], Wm_abc4/1  "Wm_abc"
  BLDC abc model4/1(dX) -> Integrator3/1
  ParkClarke4/1(Y_dq) -> Unit Delay2/1
  Constant7/1 -> Add8/1  "i_d_ref"
  PID Controller7/1 -> Add9/1  "i_q_ref"
  [Theta_abc_4] -> ParkClarke4/2(theta)
  Add8/1 -> PID Controller9/1
  Add9/1 -> PID Controller8/1
  PID Controller9/1 -> Mux3/1
  Unit Delay2/1 -> Demux3/1
  Integrator3/1 -> Graphs4/1(X), BLDC abc model4/1(X), Fases abc4/1(X)
  Add7/1 -> PID Controller7/1
  [Wm_abc_4] -> Add7/2
  PID Controller8/1 -> Mux3/2
  Demux3/1 -> Add8/2
  Mux3/1 -> InvPark/1(X_dq)
  [Theta_abc_4] -> InvPark/2(theta)
  Demux/1 -> MATLAB Function/1(x)
  Demux/2 -> MATLAB Function/2(y)
  MATLAB Function/1(r) -> [SVPWM_Vs]
  MATLAB Function/2(theta) -> [SVPWM_theta]
  Demux/3 -> Terminator/1
  InvPark/1(Y_ab0) -> Demux/1
  Voltage Measurement1/4(Van) -> Mux/3, Phase Voltages1/1
  Space Vector calculator/2(v) -> SVPWM Generator/2(v)
  Demux4/2 -> Cast To Boolean1/1
  [Vg4] -> Mosfet3/1
  Logical Operator/1 -> [Vg2]
  Cast To Boolean/1 -> Logical Operator/1, [Vg1]
  Logical Operator1/1 -> [Vg4]
  [SVPWM_Vs] -> Space Vector calculator/2(Vs)
  Constant9/1 -> SVPWM Generator/3(Tz)
  Demux4/3 -> Cast To Boolean2/1
  SVPWM Generator/1(y) -> Demux4/1
  Voltage Measurement1/5(Vbn) -> Mux/2, Phase Voltages1/2
  Cast To Boolean1/1 -> Logical Operator1/1, [Vg3]
  [Vg1] -> Mosfet4/1
  Constant/1 -> Space Vector calculator/1(V_link)
  Cast To Boolean2/1 -> Logical Operator2/1, [Vg5]
  Demux4/1 -> Cast To Boolean/1
  Voltage Measurement1/3(Vca) -> Line Voltages1/3
  Logical Operator2/1 -> [Vg6]
  [Vg5] -> Mosfet1/1
  [Vg3] -> Mosfet2/1
  Voltage Measurement1/2(Vbc) -> Line Voltages1/2
  [SVPWM_theta] -> Space Vector calculator/3(theta_vs1)
  Voltage Measurement1/6(Vcn) -> Mux/1, Phase Voltages1/3
  Voltage Measurement1/1(Vab) -> Line Voltages1/1
  [Vg6] -> Mosfet/1
  Mux/1 -> [V_abc]
  [Vg2] -> Mosfet5/1
  Space Vector calculator/1(n) -> SVPWM Generator/1(n)
  [V_abc] -> BLDC abc model4/3(v)
  [Wm_abc_3] -> Wm_abc_comp/1  "Wm_Analysis"
  [Wm_abc_4] -> Wm_abc_comp/2  "Wm_SVPWM"
  connections:
  Mosfet2/RConn1 -- Voltage Measurement1/LConn2 -- Mosfet3/LConn1
  Mosfet/RConn1 -- Mosfet3/RConn1 -- Mosfet5/RConn1 -- DC Voltage Source/LConn1
  Mosfet2/LConn1 -- Mosfet1/LConn1 -- DC Voltage Source/RConn1 -- Mosfet4/LConn1
  Mosfet4/RConn1 -- Mosfet5/LConn1 -- Voltage Measurement1/LConn1
  Mosfet1/RConn1 -- Voltage Measurement1/LConn3 -- Mosfet/LConn1

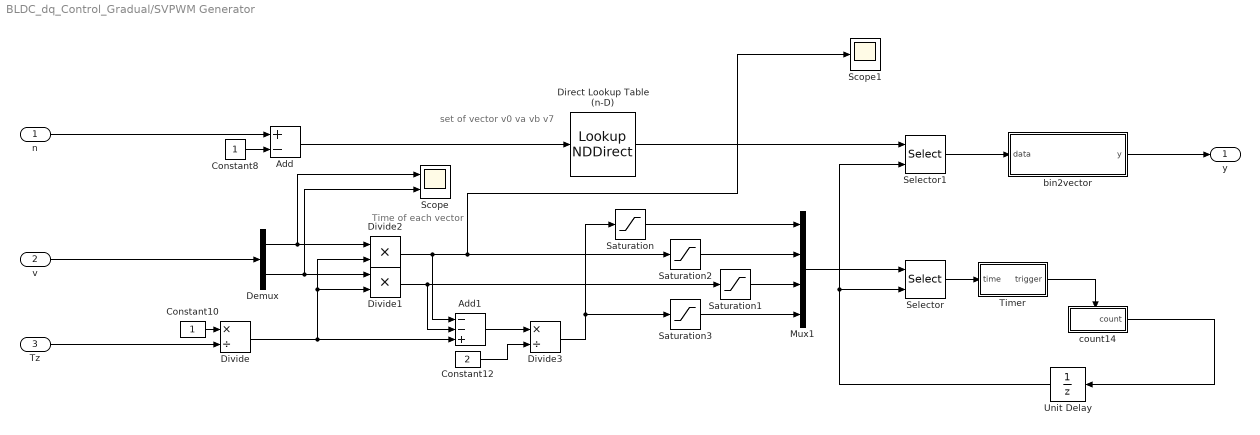
== system BLDC_dq_Control_Gradual/SVPWM Generator ==
  note: set of vector v0 va vb v7
  note: Time of each vector
  n : Inport
  v : Inport  Port=2
  Tz : Inport  Port=3
  Add : Sum  Inputs=+-
  Add1 : Sum  Inputs=--+
  Constant10 : Constant
  Constant12 : Constant  Value=2
  Constant8 : Constant
  Demux : Demux  Outputs=2
  Direct Lookup Table (n-D) : LookupNDDirect  InputsSelectThisObjectFromTable=Vector  Table=[0 1 3 7;0 3 2 7;0 2 6 7;0 6 4 7; 0 4 5 7;0 5 1 7]'
  Divide : Product  Inputs=*/
  Divide1 : Product  Inputs=**
  Divide2 : Product  Inputs=**
  Divide3 : Product  Inputs=*/
  Mux1 : Mux
  Saturation{,1..3} (4 alike) : Saturate  UpperLimit=10000000  LowerLimit=0.00005
  Scope : Scope  NumInputPorts=2
  Scope1 : Scope
  Selector : Selector  InputPortWidth=4  IndexOptions=Index vector (port)  Indices=[1 3]  OutputSizes=1
  Selector1 : Selector  InputPortWidth=4  IndexOptions=Index vector (port)  Indices=[1 3]  OutputSizes=1
  Timer : Subsystem
  Unit Delay : UnitDelay  InitialCondition=1  SampleTime=-1  HasFrameUpgradeWarning=on
  bin2vector : MATLAB Function  TreatAsAtomicUnit=on
  count14 : Subsystem  TreatAsAtomicUnit=on
  y : Outport
  wires:
  Constant10/1 -> Divide/1
  Divide3/1 -> Saturation3/1, Saturation/1
  Divide1/1 -> Add1/2, Saturation1/1
  Constant8/1 -> Add/2
  v/1 -> Demux/1
  Divide2/1 -> Add1/1, Scope1/1, Saturation2/1
  Add/1 -> Direct Lookup Table (n-D)/1
  Divide/1 -> Divide1/2, Divide2/2, Add1/3
  count14/1(count) -> Unit Delay/1
  bin2vector/1(y) -> y/1
  Add1/1 -> Divide3/1
  Demux/2 -> Scope/2, Divide1/1
  Direct Lookup Table (n-D)/1 -> Selector1/1
  Demux/1 -> Scope/1, Divide2/1
  Constant12/1 -> Divide3/2
  Mux1/1 -> Selector/1
  n/1 -> Add/1
  Unit Delay/1 -> Selector1/2, Selector/2
  Selector/1 -> Timer/1(time)
  Timer/1(trigger) -> count14/Trigger
  Selector1/1 -> bin2vector/1(data)
  Tz/1 -> Divide/2
  Saturation/1 -> Mux1/1
  Saturation3/1 -> Mux1/4
  Saturation1/1 -> Mux1/3
  Saturation2/1 -> Mux1/2

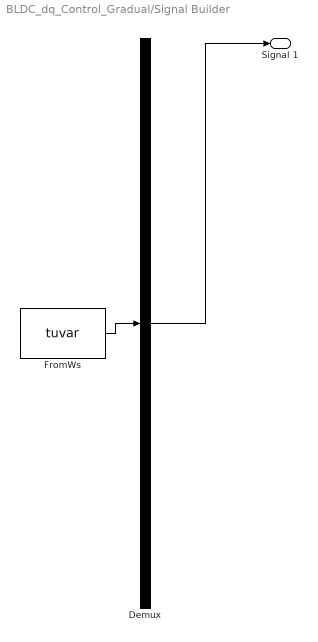
== system BLDC_dq_Control_Gradual/Signal Builder ==
  Demux : Demux  Tag=STV Demux  Outputs=1
      settings: DisplayOption=none
  FromWs : FromWorkspace  Tag=STV FromWs  VariableName=tuvar
      SigBuilderData=|
      | common.afterFinalStr = 'Extrapolate'
      | common.sampleTime = 0
      | dataSet.timeRange = [0 30]
      | dataSet.name = 'Group 1'
      | sbobj.Groups.Name = 'Group 1'
      | sbobj.Groups.Signals.Name = 'Signal 1'
      | sbobj.Groups.Signals.XData = [0 4 4 6 6 10 30]
      | sbobj.Groups.Signals.YData = [8.05 8.05 20 20 15 4 4]
      | sbobj.Groups.TimeRange = [0 30]
  Signal 1 : Outport  Tag=STV Outport
  wires:
  Demux/1 -> Signal 1/1
  FromWs/1 -> Demux/1

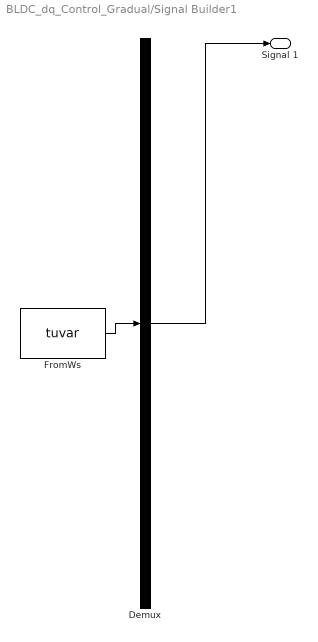
== system BLDC_dq_Control_Gradual/Signal Builder1 ==
  Demux : Demux  Tag=STV Demux  Outputs=1
      settings: DisplayOption=none
  FromWs : FromWorkspace  Tag=STV FromWs  VariableName=tuvar
      SigBuilderData=|
      | common.afterFinalStr = 'Extrapolate'
      | common.sampleTime = 0
      | dataSet.timeRange = [0 30]
      | dataSet.name = 'Group 1'
      | sbobj.Groups.Name = 'Group 1'
      | sbobj.Groups.Signals.Name = 'Signal 1'
      | sbobj.Groups.Signals.XData = [0 4 4 6 6 10 30]
      | sbobj.Groups.Signals.YData = [8.05 8.05 20 20 15 4 4]
      | sbobj.Groups.TimeRange = [0 30]
  Signal 1 : Outport  Tag=STV Outport
  wires:
  Demux/1 -> Signal 1/1
  FromWs/1 -> Demux/1

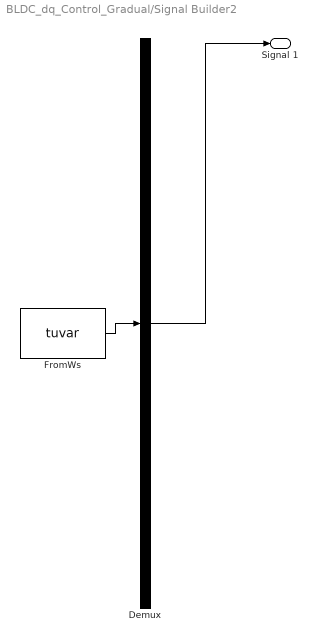
== system BLDC_dq_Control_Gradual/Signal Builder2 ==
  Demux : Demux  Tag=STV Demux  Outputs=1
      settings: DisplayOption=none
  FromWs : FromWorkspace  Tag=STV FromWs  VariableName=tuvar
      SigBuilderData=|
      | common.afterFinalStr = 'Extrapolate'
      | common.sampleTime = 0
      | dataSet.timeRange = [0 30]
      | dataSet.name = 'Group 1'
      | sbobj.Groups.Name = 'Group 1'
      | sbobj.Groups.Signals.Name = 'Signal 1'
      | sbobj.Groups.Signals.XData = [0 4 4 6 6 10 30]
      | sbobj.Groups.Signals.YData = [8.05 8.05 20 20 15 4 4]
      | sbobj.Groups.TimeRange = [0 30]
  Signal 1 : Outport  Tag=STV Outport
  wires:
  Demux/1 -> Signal 1/1
  FromWs/1 -> Demux/1

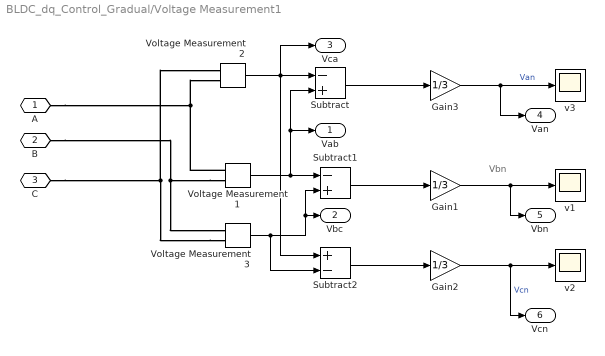
== system BLDC_dq_Control_Gradual/Voltage Measurement1 ==
  note: Vbn
  Gain1 : Gain  Gain=1/3
  Gain2 : Gain  Gain=1/3
  Gain3 : Gain  Gain=1/3
  Subtract : Sum  Inputs=-+
  Subtract1 : Sum  Inputs=-+
  Subtract2 : Sum  Inputs=+-
  Voltage Measurement1 : spsVoltageMeasurementLib/Voltage Measurement  PhasorSimulation=off  OutputType=Complex  PSBequivalent=0
  Voltage Measurement2 : spsVoltageMeasurementLib/Voltage Measurement  PhasorSimulation=off  OutputType=Complex  PSBequivalent=0
  Voltage Measurement3 : spsVoltageMeasurementLib/Voltage Measurement  PhasorSimulation=off  OutputType=Complex  PSBequivalent=0
  v1 : Scope
  v2 : Scope
  v3 : Scope
  A : PMIOPort  Side=Left
  B : PMIOPort  Port=2  Side=Left
  C : PMIOPort  Port=3  Side=Left
  Vab : Outport  VectorParamsAs1DForOutWhenUnconnected=off
  Vbc : Outport  Port=2  VectorParamsAs1DForOutWhenUnconnected=off
  Vca : Outport  Port=3  VectorParamsAs1DForOutWhenUnconnected=off
  Van : Outport  Port=4  VectorParamsAs1DForOutWhenUnconnected=off
  Vbn : Outport  Port=5  VectorParamsAs1DForOutWhenUnconnected=off
  Vcn : Outport  Port=6  VectorParamsAs1DForOutWhenUnconnected=off
  wires:
  Gain2/1 -> v2/1, Vcn/1  "Vcn"
  Subtract2/1 -> Gain2/1
  Gain1/1 -> v1/1, Vbn/1
  Subtract1/1 -> Gain1/1
  Voltage Measurement3/1 -> Subtract1/2, Vbc/1, Subtract2/2
  Gain3/1 -> v3/1, Van/1  "Van"
  Subtract/1 -> Gain3/1
  Voltage Measurement1/1 -> Vab/1, Subtract/2, Subtract1/1
  Voltage Measurement2/1 -> Vca/1, Subtract2/1, Subtract/1
  connections:
  Voltage Measurement1/LConn1 -- A/RConn1 -- Voltage Measurement2/LConn2
  Voltage Measurement1/LConn2 -- B/RConn1 -- Voltage Measurement3/LConn1
  Voltage Measurement3/LConn2 -- Voltage Measurement2/LConn1 -- C/RConn1

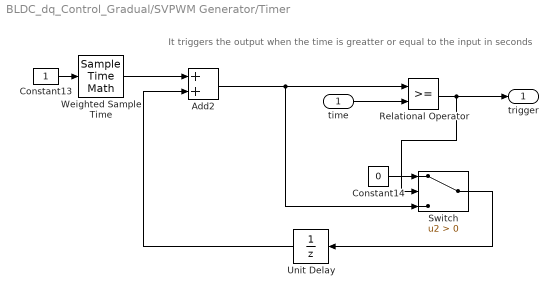
== system BLDC_dq_Control_Gradual/SVPWM Generator/Timer ==
  note: It triggers the output when the time is greatter or equal to the input in seconds
  time : Inport
  Add2 : Sum
  Constant13 : Constant
  Constant14 : Constant  Value=0
  Relational Operator : RelationalOperator  OutDataTypeStr=boolean  RndMeth=Simplest
  Switch : Switch  Criteria=u2 > Threshold
  Unit Delay : UnitDelay  SampleTime=-1  HasFrameUpgradeWarning=on
  Weighted Sample Time : SampleTimeMath  TsampMathOp=Ts Only
  trigger : Outport
  wires:
  Switch/1 -> Unit Delay/1
  Add2/1 -> Relational Operator/1, Switch/3
  Relational Operator/1 -> trigger/1, Switch/2
  Weighted Sample Time/1 -> Add2/1
  Constant13/1 -> Weighted Sample Time/1
  Constant14/1 -> Switch/1
  Unit Delay/1 -> Add2/2
  time/1 -> Relational Operator/2

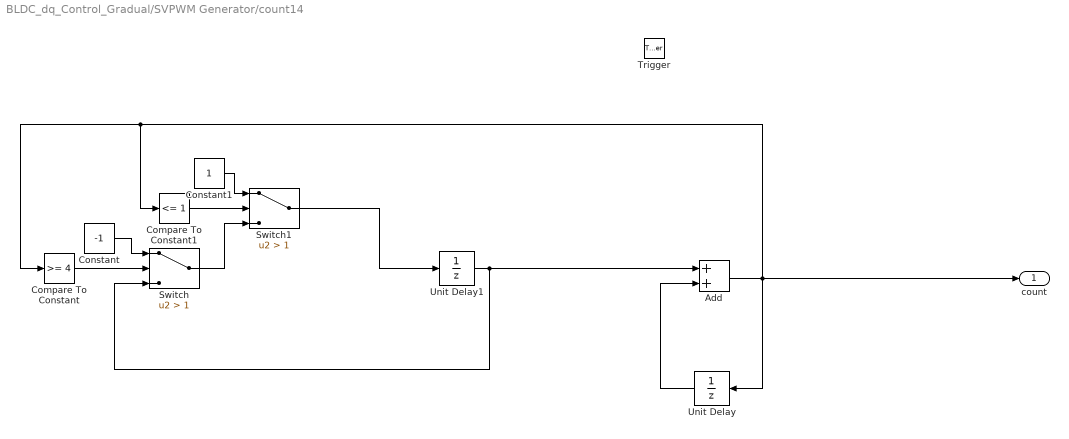
== system BLDC_dq_Control_Gradual/SVPWM Generator/count14 ==
  Trigger : TriggerPort  VariantControl=(inherit)
  Add : Sum
  Compare To Constant : simulink/Logic and Bit Operations/Compare To Constant  relop=>=  const=4  OutDataTypeStr=boolean
  Compare To Constant1 : simulink/Logic and Bit Operations/Compare To Constant  relop=<=  const=1  OutDataTypeStr=boolean
  Constant : Constant  Value=-1
  Constant1 : Constant
  Switch : Switch  Criteria=u2 > Threshold  Threshold=1
  Switch1 : Switch  Criteria=u2 > Threshold  Threshold=1
  Unit Delay : UnitDelay  InitialCondition=1  SampleTime=-1  HasFrameUpgradeWarning=on
  Unit Delay1 : UnitDelay  InitialCondition=1  SampleTime=-1  HasFrameUpgradeWarning=on
  count : Outport  InitialOutput=1
  wires:
  Add/1 -> Unit Delay/1, count/1, Compare To Constant/1, Compare To Constant1/1
  Unit Delay/1 -> Add/2
  Unit Delay1/1 -> Switch/3, Add/1
  Constant/1 -> Switch/1
  Switch/1 -> Switch1/3
  Switch1/1 -> Unit Delay1/1
  Compare To Constant/1 -> Switch/2
  Compare To Constant1/1 -> Switch1/2
  Constant1/1 -> Switch1/1

== matlab function BLDC_dq_Control_Gradual/BLDC dq model ==
  data: X input; f input; v input; dX output; Tl input
function dX = fcn(X,f,v,Tl)
i_d = X(1); i_q = X(2); wm = X(3); theta = X(4);
i_dq = X(1:2);

lambda = 0.0433; %
R = 0.35;    %ohms armature resistance
L = 0.001;  %H armature inductance
M = 0.0000;  %H mutual inductance
J = 0.00018; % kgm^2 motor inertia
P = 4; % number of poles
b = 0.0034;    %Nms Hydraulic friction coefficient of motor rotor


M_LR = [-R/(L-M)  wm; -wm  -R/(L-M)];                
                
% Park clarke transform eliminating the third element
PC_Te = (sqrt(2)/2)*[sqrt(3)*cos(theta)  sin(theta)  -sin(theta) ; ...
                    -sqrt(3)*sin(theta)  cos(theta)  -cos(theta)];

PC_T = PC_Te;

e_dq =(lambda*wm)*PC_Te*f;

v_dq = v;

di_dq = M_LR*i_dq + (1/(L-M))*v_dq - (1/(L-M))*e_dq;
T_e = (e_dq'*i_dq)/wm;
dwm = (T_e - Tl -b*wm)/J;
dtheta = (P/2)*wm;

dX = [di_dq;dwm;dtheta];

end

== matlab function BLDC_dq_Control_Gradual/Phases abc ==
  data: X input; Fabc output
function Fabc = fcn(X)
Fabc = [0;0;0];
    theta = mod(X(4),2*pi); %X(4)
    %theta = mod(X,2*pi);
    
    if (0<=theta)&&(theta<(pi/6))
        Fa = (6/pi)*theta;
    elseif ((pi/6)<=theta)&&(theta<(5*pi/6))
        Fa = 1;
    elseif ((5*pi/6<=theta))&&(theta<(7*pi/6))
        Fa = (6/pi)*(pi-theta);
    elseif ((7*pi/6)<=theta)&&(theta<(11*pi/6))
        Fa = -1;
    elseif ((11*pi/6)<=theta)&&(theta<(2*pi))
        Fa = (6/pi)*(theta-2*pi);
    else
        Fa = NaN;
    end
    
    if (0<=theta)&&(theta<(3*pi/6))
        Fb = -1;
    elseif ((3*pi/6)<=theta)&&(theta<(5*pi/6))
        Fb = (6/pi)*(theta-(2*pi)/3);
    elseif ((5*pi/6)<=theta)&&(theta<(9*pi/6))
        Fb = 1;
    elseif ((9*pi/6)<=theta)&&(theta<(11*pi/6))
        Fb = (6/pi)*(-theta+(5*pi)/3);
    elseif ((11*pi/6)<=theta)&&(theta<(2*pi))
        Fb = -1;
    else
        Fb = NaN;
    end
    
    if (0<=theta)&&(theta<(pi/6))
        Fc = 1;
    elseif ((pi/6)<=theta)&&(theta<(3*pi/6))
        Fc = (6/pi)*(pi/3-theta);
    elseif ((3*pi/6)<=theta)&&(theta<(7*pi/6))
        Fc = -1;
    elseif ((7*pi/6)<=theta)&&(theta<(9*pi/6))
        Fc = (6/pi)*(theta-(4*pi)/3);
    elseif ((9*pi/6)<=theta)&&(theta<(2*pi))
        Fc = 1;
    else
        Fc = NaN; 
    end
        
     Fa = sin(theta);
     Fb = sin(theta - 2*pi/3);
     Fc = sin(theta + 2*pi/3);
    
    Fabc = [Fa;Fb;Fc];
end

== matlab function BLDC_dq_Control_Gradual/Graphs ==
  data: X input; theta output; Wm output; Idq output
function [theta,Wm,Idq] = DEMUX(X)
theta = X(4); Wm = X(3);Idq = X(1:2);

== matlab function BLDC_dq_Control_Gradual/BLDC abc model4 ==
  data: X input; f input; v input; dX output; Tl input
function dX = fcn(X,f,v,Tl)
u = [v;Tl]; 
i_a = X(1); i_b = X(2); i_c = X(3); wm = X(4); theta = X(5);

lambda = 0.0433; %
R = 0.35;    %ohms armature resistance
L = 0.001;  %H armature inductance
M = 0.0000;  %H mutual inductance
J = 0.00018; % kgm^2 motor inertia
P = 4; % number of poles
b = 0.0034;    %Nms Hydraulic friction coefficient of motor rotor

%e = [(lamda*wm).*f;0;0];

A =[-(R/(L-M)) 0 0 -(lambda/(L-M))*f(1) 0;...
    0 -(R/(L-M)) 0 -(lambda/(L-M))*f(2) 0;...
    0 0 -(R/(L-M)) -(lambda/(L-M))*f(3) 0;...
    (lambda/J)*f(1) (lambda/J)*f(2) (lambda/J)*f(3) -b/J 0;...
    0 0 0 P/2 0];

B = diag([1/(L-M) 1/(L-M) 1/(L-M) -1/J]);
B = [B;0 0 0 0];


dX = [0;0;0;0;0];
dX = A*X + B*u;

end

== matlab function BLDC_dq_Control_Gradual/Fases abc4 ==
  data: X input; Fabc output
function Fabc = fcn(X)
Fabc = [0;0;0];
    theta = mod(X(5),2*pi); %X(4)
    %theta = mod(X,2*pi);
    
    if (0<=theta)&&(theta<(pi/6))
        Fa = (6/pi)*theta;
    elseif ((pi/6)<=theta)&&(theta<(5*pi/6))
        Fa = 1;
    elseif ((5*pi/6<=theta))&&(theta<(7*pi/6))
        Fa = (6/pi)*(pi-theta);
    elseif ((7*pi/6)<=theta)&&(theta<(11*pi/6))
        Fa = -1;
    elseif ((11*pi/6)<=theta)&&(theta<(2*pi))
        Fa = (6/pi)*(theta-2*pi);
    else
        Fa = NaN;
    end
    
    if (0<=theta)&&(theta<(3*pi/6))
        Fb = -1;
    elseif ((3*pi/6)<=theta)&&(theta<(5*pi/6))
        Fb = (6/pi)*(theta-(2*pi)/3);
    elseif ((5*pi/6)<=theta)&&(theta<(9*pi/6))
        Fb = 1;
    elseif ((9*pi/6)<=theta)&&(theta<(11*pi/6))
        Fb = (6/pi)*(-theta+(5*pi)/3);
    elseif ((11*pi/6)<=theta)&&(theta<(2*pi))
        Fb = -1;
    else
        Fb = NaN;
    end
    
    if (0<=theta)&&(theta<(pi/6))
        Fc = 1;
    elseif ((pi/6)<=theta)&&(theta<(3*pi/6))
        Fc = (6/pi)*(pi/3-theta);
    elseif ((3*pi/6)<=theta)&&(theta<(7*pi/6))
        Fc = -1;
    elseif ((7*pi/6)<=theta)&&(theta<(9*pi/6))
        Fc = (6/pi)*(theta-(4*pi)/3);
    elseif ((9*pi/6)<=theta)&&(theta<(2*pi))
        Fc = 1;
    else
        Fc = NaN; 
    end
    
    
%     
     Fa = sin(theta);
     Fb = sin(theta - 2*pi/3);
     Fc = sin(theta + 2*pi/3);
    
    Fabc = [Fa;Fb;Fc];
end

== matlab function BLDC_dq_Control_Gradual/Graphs4 ==
  data: X input; theta output; Wm output; Iabc output
function [theta,Wm,Iabc] = DEMUX(X)
theta = X(5); Wm = X(4);Iabc = X(1:3);

== matlab function BLDC_dq_Control_Gradual/MATLAB Function ==
  data: r output; x input; theta output; y input
function [r, theta] = rec2polar(x, y)

r = sqrt(x^2 + y^2);
theta = atan2(y,x);

== matlab function BLDC_dq_Control_Gradual/ParkClarke4 ==
  data: X_abc input; Y_dq output; theta input
function Y_dq = fcn(X_abc, theta)

% Park clarke transform eliminating the third element
PC_T = (sqrt(2)/2)*[sqrt(3)*cos(theta)  sin(theta)  -sin(theta) ; ...
                    -sqrt(3)*sin(theta)  cos(theta)  -cos(theta)];

Y_dq =PC_T*X_abc;
end

== matlab function BLDC_dq_Control_Gradual/InvPark ==
  data: X_dq input size=[2 1]; Y_ab0 output; theta input
function Y_ab0 = fcn(X_dq, theta)
X_dq0 = [X_dq; 0];

%inverse Park 
iT_C = [cos(theta)   -sin(theta)    0; ...
        sin(theta)    cos(theta)    0; ...
        0             0             1];
%               
             
Y_ab0 =iT_C*X_dq0;
end

== matlab function BLDC_dq_Control_Gradual/SVPWM Generator/bin2vector ==
  data: y output; data input
function y = binary2vector(data)
y = [0; 0; 0];
g = dec2bin(data,3);
out = g-'0';
y(1) = out(1);
y(2) = out(2);
y(3) = out(3);


% powOf2 = 2.^[0:nBits-1];
% 
% %# do a tiny bit of error-checking
% if data > sum(powOf2)
%    error('not enough bits to represent the data')
% end
% 
% out = false(1,nBits);
% 
% ct = nBits;
% 
% while data>0
% if data >= powOf2(ct)
% data = data-powOf2(ct);
% out(ct) = true;
% end
% ct = ct - 1;
% end

== matlab function BLDC_dq_Control_Gradual/Space Vector calculator ==
  data: n output; v output; theta_vs output; V_link input; Vs input; theta_vs1 input
function [n,v,theta_vs]= SpaceVectorCalc(V_link,Vs,theta_vs1)
v = [0 0];
theta_vs = mod(theta_vs1,2*pi);
theta = 0;
n = 0; % This is the quadrant of the vector. you should never get zero as output

if 0*(pi/180) <= theta_vs && theta_vs < 60*(pi/180)
   theta = theta_vs;
   n = 1;
elseif 60*(pi/180) <= theta_vs && theta_vs < 120*(pi/180)
   theta = theta_vs - 60*(pi/180);
   n = 2;
elseif 120*(pi/180) <= theta_vs && theta_vs < 180*(pi/180)  
    theta = theta_vs - 2*60*(pi/180);
    n = 3;
elseif 180*(pi/180) <= theta_vs && theta_vs < 240*(pi/180)  
    theta = theta_vs - 3*60*(pi/180);
    n = 4;
elseif 240*(pi/180) <= theta_vs && theta_vs < 300*(pi/180)
    theta = theta_vs - 4*60*(pi/180);
    n = 5;
elseif 300*(pi/180) <= theta_vs && theta_vs < 360*(pi/180)
    theta = theta_vs - 5*60*(pi/180);
    n = 6;
end


V_b = ((2*Vs)/sqrt(3))*sin(theta);
V_a = ((2*Vs)/sqrt(3))*sin(pi/3 - theta);

v = [V_a V_b];

== matlab function BLDC_dq_Control_Gradual/BLDC abc model1 ==
  data: X input; f input; v input; dX output; Tl input
function dX = fcn(X,f,v,Tl)
u = [v;Tl]; 
i_a = X(1); i_b = X(2); i_c = X(3); wm = X(4); theta = X(5);

lambda = 0.0433; %
R = 0.35;    %ohms armature resistance
L = 0.001;  %H armature inductance
M = 0.0000;  %H mutual inductance
J = 0.00018; % kgm^2 motor inertia
P = 4; % number of poles
b = 0.0034;    %Nms Hydraulic friction coefficient of motor rotor

%e = [(lamda*wm).*f;0;0];

A =[-(R/(L-M)) 0 0 -(lambda/(L-M))*f(1) 0;...
    0 -(R/(L-M)) 0 -(lambda/(L-M))*f(2) 0;...
    0 0 -(R/(L-M)) -(lambda/(L-M))*f(3) 0;...
    (lambda/J)*f(1) (lambda/J)*f(2) (lambda/J)*f(3) -b/J 0;...
    0 0 0 P/2 0];

B = diag([1/(L-M) 1/(L-M) 1/(L-M) -1/J]);
B = [B;0 0 0 0];


dX = [0;0;0;0;0];
dX = A*X + B*u;

end

== matlab function BLDC_dq_Control_Gradual/Fases abc1 ==
  data: X input; Fabc output
function Fabc = fcn(X)
Fabc = [0;0;0];
    theta = mod(X(5),2*pi); %X(4)
    %theta = mod(X,2*pi);
    
    if (0<=theta)&&(theta<(pi/6))
        Fa = (6/pi)*theta;
    elseif ((pi/6)<=theta)&&(theta<(5*pi/6))
        Fa = 1;
    elseif ((5*pi/6<=theta))&&(theta<(7*pi/6))
        Fa = (6/pi)*(pi-theta);
    elseif ((7*pi/6)<=theta)&&(theta<(11*pi/6))
        Fa = -1;
    elseif ((11*pi/6)<=theta)&&(theta<(2*pi))
        Fa = (6/pi)*(theta-2*pi);
    else
        Fa = NaN;
    end
    
    if (0<=theta)&&(theta<(3*pi/6))
        Fb = -1;
    elseif ((3*pi/6)<=theta)&&(theta<(5*pi/6))
        Fb = (6/pi)*(theta-(2*pi)/3);
    elseif ((5*pi/6)<=theta)&&(theta<(9*pi/6))
        Fb = 1;
    elseif ((9*pi/6)<=theta)&&(theta<(11*pi/6))
        Fb = (6/pi)*(-theta+(5*pi)/3);
    elseif ((11*pi/6)<=theta)&&(theta<(2*pi))
        Fb = -1;
    else
        Fb = NaN;
    end
    
    if (0<=theta)&&(theta<(pi/6))
        Fc = 1;
    elseif ((pi/6)<=theta)&&(theta<(3*pi/6))
        Fc = (6/pi)*(pi/3-theta);
    elseif ((3*pi/6)<=theta)&&(theta<(7*pi/6))
        Fc = -1;
    elseif ((7*pi/6)<=theta)&&(theta<(9*pi/6))
        Fc = (6/pi)*(theta-(4*pi)/3);
    elseif ((9*pi/6)<=theta)&&(theta<(2*pi))
        Fc = 1;
    else
        Fc = NaN; 
    end
    
    
%     
     Fa = sin(theta);
     Fb = sin(theta - 2*pi/3);
     Fc = sin(theta + 2*pi/3);
    
    Fabc = [Fa;Fb;Fc];
end

== matlab function BLDC_dq_Control_Gradual/Fases abc3 ==
  data: X input; Fabc output
function Fabc = fcn(X)
Fabc = [0;0;0];
    theta = mod(X(5),2*pi); %X(4)
    %theta = mod(X,2*pi);
    
    if (0<=theta)&&(theta<(pi/6))
        Fa = (6/pi)*theta;
    elseif ((pi/6)<=theta)&&(theta<(5*pi/6))
        Fa = 1;
    elseif ((5*pi/6<=theta))&&(theta<(7*pi/6))
        Fa = (6/pi)*(pi-theta);
    elseif ((7*pi/6)<=theta)&&(theta<(11*pi/6))
        Fa = -1;
    elseif ((11*pi/6)<=theta)&&(theta<(2*pi))
        Fa = (6/pi)*(theta-2*pi);
    else
        Fa = NaN;
    end
    
    if (0<=theta)&&(theta<(3*pi/6))
        Fb = -1;
    elseif ((3*pi/6)<=theta)&&(theta<(5*pi/6))
        Fb = (6/pi)*(theta-(2*pi)/3);
    elseif ((5*pi/6)<=theta)&&(theta<(9*pi/6))
        Fb = 1;
    elseif ((9*pi/6)<=theta)&&(theta<(11*pi/6))
        Fb = (6/pi)*(-theta+(5*pi)/3);
    elseif ((11*pi/6)<=theta)&&(theta<(2*pi))
        Fb = -1;
    else
        Fb = NaN;
    end
    
    if (0<=theta)&&(theta<(pi/6))
        Fc = 1;
    elseif ((pi/6)<=theta)&&(theta<(3*pi/6))
        Fc = (6/pi)*(pi/3-theta);
    elseif ((3*pi/6)<=theta)&&(theta<(7*pi/6))
        Fc = -1;
    elseif ((7*pi/6)<=theta)&&(theta<(9*pi/6))
        Fc = (6/pi)*(theta-(4*pi)/3);
    elseif ((9*pi/6)<=theta)&&(theta<(2*pi))
        Fc = 1;
    else
        Fc = NaN; 
    end
    
    
%     
     Fa = sin(theta);
     Fb = sin(theta - 2*pi/3);
     Fc = sin(theta + 2*pi/3);
    
    Fabc = [Fa;Fb;Fc];
end

== matlab function BLDC_dq_Control_Gradual/BLDC abc model ==
  data: X input; f input; v input; dX output; Tl input
function dX = fcn(X,f,v,Tl)
u = [v;Tl]; 
i_a = X(1); i_b = X(2); i_c = X(3); wm = X(4); theta = X(5);

lambda = 0.0433; %
R = 0.35;    %ohms armature resistance
L = 0.001;  %H armature inductance
M = 0.0000;  %H mutual inductance
J = 0.00018; % kgm^2 motor inertia
P = 4; % number of poles
b = 0.0034;    %Nms Hydraulic friction coefficient of motor rotor

%e = [(lamda*wm).*f;0;0];

A =[-(R/(L-M)) 0 0 -(lambda/(L-M))*f(1) 0;...
    0 -(R/(L-M)) 0 -(lambda/(L-M))*f(2) 0;...
    0 0 -(R/(L-M)) -(lambda/(L-M))*f(3) 0;...
    (lambda/J)*f(1) (lambda/J)*f(2) (lambda/J)*f(3) -b/J 0;...
    0 0 0 P/2 0];

B = diag([1/(L-M) 1/(L-M) 1/(L-M) -1/J]);
B = [B;0 0 0 0];


dX = [0;0;0;0;0];
dX = A*X + B*u;

end

== matlab function BLDC_dq_Control_Gradual/Gráficas2 ==
  data: X input; theta output; Wm output; Iabc output
function [theta,Wm,Iabc] = DEMUX(X)
theta = X(5); Wm = X(4);Iabc = X(1:3);

== matlab function BLDC_dq_Control_Gradual/Gráficas1 ==
  data: X input; theta output; Wm output; Iabc output
function [theta,Wm,Iabc] = DEMUX(X)
theta = X(5); Wm = X(4);Iabc = X(1:3);

== matlab function BLDC_dq_Control_Gradual/InvParkClarke ==
  data: X_dq input; Y_abc output; theta input
function Y_abc = fcn(X_dq, theta)
X_dq0 = [X_dq;0];

%inverse Park-Clarke power invariant
iT_PC = sqrt(2/3)*[cos(theta)          -sin(theta)            1/sqrt(2); ...
                  cos(theta-2*pi/3)   -sin(theta-2*pi/3)     1/sqrt(2); ...
                  cos(theta+2*pi/3)   -sin(theta+2*pi/3)     1/sqrt(2)];
%               
              
 %inverse Park-Clarke amplitude invariant
% iT_PC = [cos(theta)          -sin(theta)            1; ...
%          cos(theta-2*pi/3)   -sin(theta-2*pi/3)     1; ...
%          cos(theta+2*pi/3)   -sin(theta+2*pi/3)     1];



Y_abc =iT_PC*X_dq0;
end
